simulink model "qs_topo3_compare"  (R2023b)
settings: Solver=ode45  StartTime=0.0  StopTime=48  MaxStep=0.1  RelTol=1e-3
InitFcn:
  | mw = get_param(bdroot,'ModelWorkspace'); evalin(mw,'xq = N_pop .* (frac_init ./ sum(frac_init));'); evalin(mw,'x0_1 = xq(1);'); evalin(mw,'x0_2 = xq(2);'); evalin(mw,'x0_3 = xq(3);');
model workspace (MAT data in the model file):
  A0 = 0
  K = 1
  KA = 0.75
  M = 3
  N_pop = 0.2
  b_vec = [0.58 0.36]
  c_signal = 4
  c_vec = [0.24 0.16]
  dA = 0.05
  decepStrength = 1
  delta_qs = 0.01
  enableFoodLimit = 1
  epsN = 1e-09
  eta_game = 0.35
  foodAccessMin = 0.1
  foodAmbient = 0.02
  frac_init = [0.333333333333 0.333333333333 0.333333333333]
  kA_vec = [0.1 0 0]
  n = 2
  nTraits = 2
  need_floor = 1e-09
  need_vec = [1 1 1]
  omega0 = 1
  produce = [1  1; 0  1; 1  0]
  qsBoost = 1
  r = 0.65
  x0_1 = 0.0666666666667
  x0_2 = 0.0666666666667
  x0_3 = 0.0666666666667
  xq = [0.0666666666667 0.0666666666667 0.0666666666667]
undefined symbols (not defined in the file or in its folder): qs_mspg_rhs_component
settings Model: Creator=14227  LastModifiedBy=14227

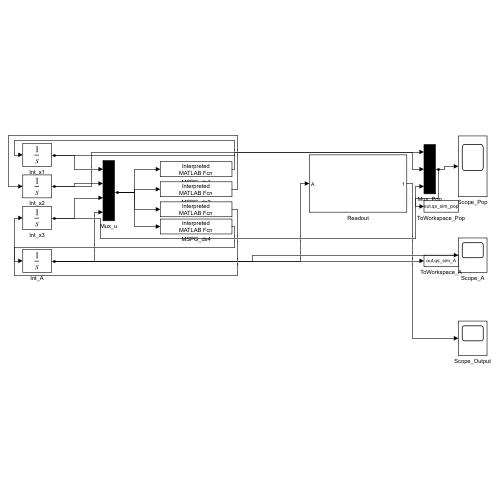
[thumbnail: Simulink's stored preview of the top-level diagram]
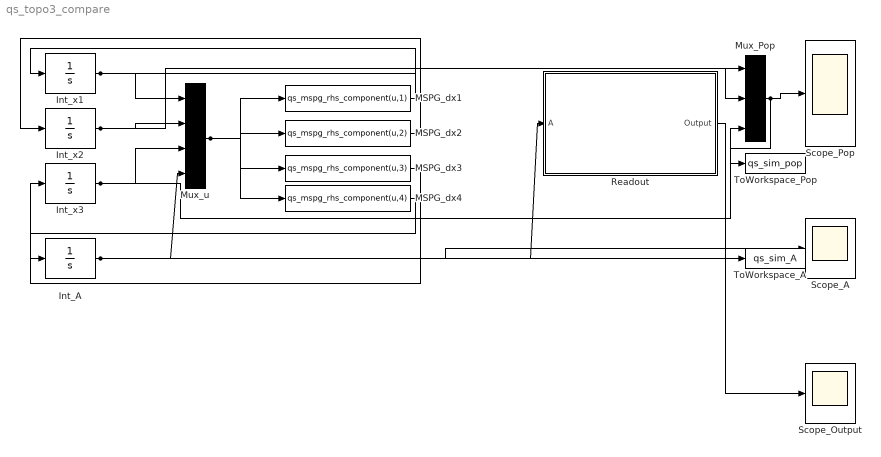
== system qs_topo3_compare ==
  Int_A : Integrator  InitialCondition=A0
  Int_x1 : Integrator  InitialCondition=x0_1
  Int_x2 : Integrator  InitialCondition=x0_2
  Int_x3 : Integrator  InitialCondition=x0_3
  MSPG_dx1 : MATLABFcn  MATLABFcn=qs_mspg_rhs_component(u,1)
  MSPG_dx2 : MATLABFcn  MATLABFcn=qs_mspg_rhs_component(u,2)
  MSPG_dx3 : MATLABFcn  MATLABFcn=qs_mspg_rhs_component(u,3)
  MSPG_dx4 : MATLABFcn  MATLABFcn=qs_mspg_rhs_component(u,4)
  Mux_Pop : Mux  Inputs=3
  Mux_u : Mux
  Readout : Subsystem
  Scope_A : Scope
  Scope_Output : Scope
  Scope_Pop : Scope
  ToWorkspace_A : ToWorkspace  VariableName=qs_sim_A  SaveFormat=Structure With Time  SampleTime=-1
  ToWorkspace_Pop : ToWorkspace  VariableName=qs_sim_pop  SaveFormat=Structure With Time  SampleTime=-1
  wires:
  Int_x1/1 -> Mux_u/1, Mux_Pop/1
  Int_x2/1 -> Mux_u/2, Mux_Pop/2
  Int_x3/1 -> Mux_u/3, Mux_Pop/3
  Int_A/1 -> Mux_u/4, Scope_A/1, Readout/1(A), ToWorkspace_A/1
  Mux_u/1 -> MSPG_dx1/1, MSPG_dx2/1, MSPG_dx3/1, MSPG_dx4/1
  MSPG_dx1/1 -> Int_x1/1
  MSPG_dx2/1 -> Int_x2/1
  MSPG_dx3/1 -> Int_x3/1
  MSPG_dx4/1 -> Int_A/1
  Mux_Pop/1 -> Scope_Pop/1, ToWorkspace_Pop/1
  Readout/1(Output) -> Scope_Output/1

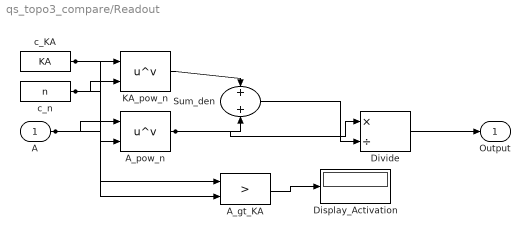
== system qs_topo3_compare/Readout ==
  A : Inport
  A_gt_KA : RelationalOperator  Operator=>  OutDataTypeStr=boolean  RndMeth=Simplest  InputSameDT=off
  A_pow_n : Math  Operator=pow
  Display_Activation : Display
  Divide : Product  Inputs=*/
  KA_pow_n : Math  Operator=pow
  Sum_den : Sum
  c_KA : Constant  Value=KA
  c_n : Constant  Value=n
  Output : Outport
  wires:
  A/1 -> A_pow_n/1, A_gt_KA/1
  c_n/1 -> A_pow_n/2, KA_pow_n/2
  c_KA/1 -> KA_pow_n/1, A_gt_KA/2
  KA_pow_n/1 -> Sum_den/1
  A_pow_n/1 -> Sum_den/2, Divide/1
  Sum_den/1 -> Divide/2
  Divide/1 -> Output/1
  A_gt_KA/1 -> Display_Activation/1
